simulink model "roll_pitch_pid_control_system1"  (R2016b)
settings: Solver=FixedStepDiscrete  StartTime=0.0  StopTime=inf  RelTol=1e-3
PostLoadFcn:
  | kFactor = 1.2;
  | 
  | KpRollAttitude = 0.630138625117681 / kFactor;
  | KiRollAttitude = 0.0552303199591522 / kFactor;
  | 
  | KpPitchAttitude = 0.630138625117681 / kFactor;
  | KiPitchAttitude = 0.0552303199591522 / kFactor;
  | 
  | KpRollRate = 1.31533836563383 / kFactor;
  | KiRollRate = 0.460338699849681 / kFactor;
  | 
  | KpPitchRate = 1.31533836563383 / kFactor;
  | KiPitchRate = 0.460338699849681 / kFactor;
  | 
  | KpYawRate = 1.31533836563383 / kFactor;
  | KiYawRate = 0.460338699849681 / kFactor;
undefined symbols (not defined in the file or in its folder): PX4_TUNE_ENUM, RGBLED_COLOR_ENUM, RGBLED_MODE_ENUM
libraries: pixhawk_slib_sensors_actuators x6, simulink x3
settings Model: SimulationMode=external  ExtModeTrigDuration=800  ExtModeArchiveFileName=EXT_mode_log  ExtModeArchiveDirName=C:\Pixhawk_Branch_Experiment\Ext_mode_bkgnd\Data_Logging  ExtModeAddSuffixToVar=on  ExtModeWriteAllDataToWs=on  ExtModeLogAll=off  Creator=Adam  LastModifiedBy=E6320
settings SolverCC: AutoInsertRateTranBlk=on
settings DataIOCC: LimitDataPoints=on  SaveFormat=Array
settings OptimizationCC: DefaultParameterBehavior=Inlined  LifeSpan=1  MaxStackSize=64
settings DebuggingCC: SolverPrmCheckMsg=warning  AllowSymbolicDim=off  SFUnexpectedBacktrackingDiag=warning  SFNoUnconditionalDefaultTransitionDiag=warning  SFExecutionAtInitializationDiag=none
settings HardwareCC: ProdBitPerPointer=32  ProdBitPerSizeT=32  ProdBitPerPtrDiffT=32  ProdLargestAtomicInteger=Long  ProdLargestAtomicFloat=Double  ProdWordSize=32  ProdHWDeviceType=ARM Compatible->ARM Cortex
settings ModelReferenceCC: PropagateSignalLabelsOutOfModel=off
settings RTWCC: SystemTargetFile=ert.tlc  HardwareBoard=Pixhawk PX4  TLCOptions=-aInlineSetEventsForThisBaseRateFcn=TLC_FALSE -aSuppressMultiTaskScheduler=TLC_FALSE -aRateBasedStepFcn=0  TemplateMakefile=ert_default_tmf  Description=Embedded Coder  GenerateReport=on  Toolchain=Pixhawk Toolchain  IncludeHyperlinkInReport=on  LaunchReport=on  GenerateTraceReport=on  GenerateTraceReportSl=on  GenerateTraceReportSf=on  GenerateTraceReportEml=on  GenerateCodeMetricsReport=on
settings CodeAppCC: IgnoreCustomStorageClasses=off
settings ERTTargetCC: CodeReplacementLibrary=GCC ARM Cortex-A9  ExtMode=on  ExtModeTransport=1  ExtModeMexFile=ext_serial_win32_comm  ExtModeMexArgs=1 7 115200 10  ERTCustomFileTemplate=PX4_codertarget_file_process.tlc  ConvertIfToSwitch=off  SuppressUnreachableDefaultCases=off
settings ConfigComp: CovMetricSettings=dw  CovHtmlReporting=on  CovSaveCumulativeToWorkspaceVar=on  CovSaveSingleToWorkspaceVar=on  CovExternalEMLEnable=off  CovSFcnEnable=off

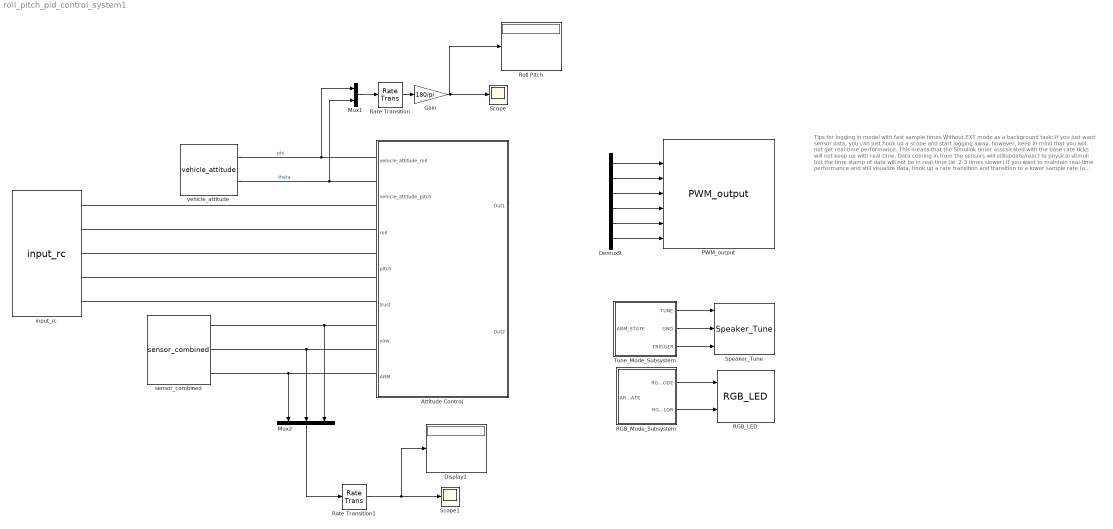
== system roll_pitch_pid_control_system1 ==
  note: Tips for logging in model with fast sample times
      |
      | Without EXT mode as a background task:
      | If you just want sensor data, you can just hook up a scope and start logging away, however, keep in mind that you will not get real-time performance. This means that the Simulink timer assosicated with the base-rate ticks will not keep up with real-time. Data coming in from the sensors will stillupdate/react to physical stimuli but the time stamp of data will not be in real-time (ie: 2-3 times slower)
      |
      | If you want to maintain real-time performance and still visualize data, hook up a rate transition and transition to a lower sample rate (a factor of 10 lower) and set the duration size to a value that will not cause the clock to slow down that much
      |
      | Recall that duration is the number of base-rate 'ticks' of data to give back. Sometimes if you set the duration too low data fails to come in for a specified sample rate. For instance, if we chose a duration value of 1:
      | 1 * 0.004 = 0.004 seconds worth of data
      | What will the lower sample (0.04s) scope show?
      | int( 0.004/0.04 ) = 0.. if we check the scope we see no data
      |
      | However, if we chose a duration value of 20
      | 400*0.004 = 1.6 seconds worth of data from base-rate
      | 1.60 / 0.04 = 40 points of data on the lower sample time scopes
      |
      | In other words, ensure the number of duration ticks gives you enough data
      | points to view on the lower sample rates, otherwise you wont see any data at all. Consult the documentation for more detail
      |
      | Using EXT mode with background task enabled
      |
      | This model has already been configured to use a background task and already uses a lot of the tips described in the above steps. With background tasking, the base-rate task is not encumbered by having to run external mode tasks at the same time, instead, EXT mode is now running in the background on another task being paced at 10 Hz. This can greatly help with real-time performance. Sometimes you may want to use the default behavior if you only have a single sample-time running at a slow rate - if you want data to come in faster or as fast as the model's sample-time then you'll want to use default behavior. On the other hand, if your model is running with multiple rates at varying speeds, you will want to pick the back-ground task option
  Attitude Control : Subsystem
  Demux9 : Demux  Outputs=6
  Display1 : Display
  Gain : Gain  Gain=180/pi
  Mux1 : Mux  Inputs=2
  Mux2 : Mux  Inputs=3
  PWM_output : pixhawk_slib_sensors_actuators/PWM_output  pwm_rate=400Hz  show_pwm1=on  show_pwm2=on  show_pwm3=on  show_pwm4=on  show_pwm5=on  show_pwm6=on  show_pwm7=off  show_pwm8=off
  RGB_LED : pixhawk_slib_sensors_actuators/RGB_LED
  RGB_Mode_Subsystem : Subsystem
  Rate Transition : RateTransition  OutPortSampleTime=0.04
  Rate Transition1 : RateTransition  OutPortSampleTime=0.04
  Roll Pitch : Display
  Scope : Scope
  Scope1 : Scope
  Speaker_Tune : pixhawk_slib_sensors_actuators/Speaker_Tune
  Tune_Mode_Subsystem : Subsystem
  input_rc : pixhawk_slib_sensors_actuators/input_rc  sampletime=1/250  channel1=on  channel2=on  channel3=on  channel4=on  channel5=on  channel6=off  channel7=off  channel8=off  ch_count=off  rssi=off  rc_failsafe=off  rc_lost=off  rc_inputsource=off
  sensor_combined : pixhawk_slib_sensors_actuators/sensor_combined  sampletime=1/250  show_mag=off  show_acc=off  show_gyro=on  show_baro=off  show_ts=off
  vehicle_attitude : pixhawk_slib_sensors_actuators/vehicle_attitude  sampletime=1/250  show_r=on  show_p=on  show_y=off  show_q=off
  wires:
  Demux9/6 -> PWM_output/7
  Demux9/5 -> PWM_output/6
  Demux9/4 -> PWM_output/5
  Demux9/2 -> PWM_output/3
  Demux9/3 -> PWM_output/4
  RGB_Mode_Subsystem/1(RGB_MODE) -> RGB_LED/1
  RGB_Mode_Subsystem/2(RGB_COLOR) -> RGB_LED/2
  Tune_Mode_Subsystem/1(TUNE) -> Speaker_Tune/1
  Tune_Mode_Subsystem/2(GND) -> Speaker_Tune/2
  Tune_Mode_Subsystem/3(TRIGGER) -> Speaker_Tune/3
  ? -> PWM_output/1, Tune_Mode_Subsystem/1(ARM_STATE), RGB_Mode_Subsystem/1(ARM_STATE)
  vehicle_attitude/1 -> Mux1/1  "phi"
  vehicle_attitude/2 -> Mux1/2  "theta"
  input_rc/1 -> ?
  input_rc/2 -> ?
  input_rc/3 -> ?
  input_rc/4 -> ?
  sensor_combined/1 -> Mux2/3
  sensor_combined/2 -> Mux2/2
  sensor_combined/3 -> Mux2/1
  ? -> Demux9/1
  Demux9/1 -> PWM_output/2
  input_rc/5 -> ?
  Mux1/1 -> Rate Transition/1
  Rate Transition/1 -> Gain/1
  Rate Transition1/1 -> Scope1/1, Display1/1
  Mux2/1 -> Rate Transition1/1
  Gain/1 -> Roll Pitch/1, Scope/1

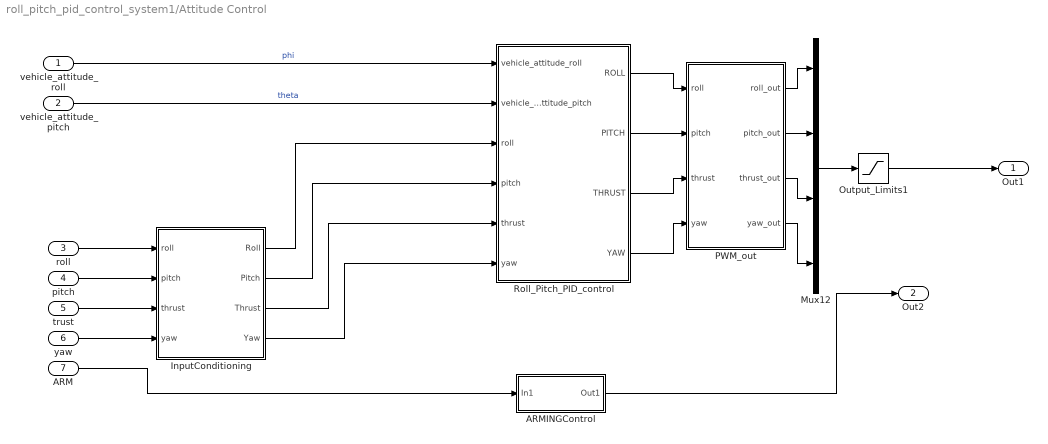
== system roll_pitch_pid_control_system1/Attitude Control ==
  vehicle_attitude_roll : Inport
  vehicle_attitude_pitch : Inport  Port=2
  roll : Inport  Port=3
  pitch : Inport  Port=4
  trust : Inport  Port=5
  yaw : Inport  Port=6
  ARM : Inport  Port=7
  ARMINGControl : Subsystem
  InputConditioning : Subsystem
  Mux12 : Mux
  Output_Limits1 : Saturate  UpperLimit=2000  LowerLimit=1000
  PWM_out : MATLAB Function  TreatAsAtomicUnit=on
  Roll_Pitch_PID_control : Subsystem
  Out1 : Outport
  Out2 : Outport  Port=2
  wires:
  vehicle_attitude_roll/1 -> Roll_Pitch_PID_control/1(vehicle_attitude_roll)  "phi"
  vehicle_attitude_pitch/1 -> Roll_Pitch_PID_control/2(vehicle_attitude_pitch)  "theta"
  ARM/1 -> ARMINGControl/1(In1)
  roll/1 -> InputConditioning/1(roll)
  pitch/1 -> InputConditioning/2(pitch)
  yaw/1 -> InputConditioning/4(yaw)
  trust/1 -> InputConditioning/3(thrust)
  ARMINGControl/1(Out1) -> Out2/1
  Output_Limits1/1 -> Out1/1
  InputConditioning/1(Roll) -> Roll_Pitch_PID_control/3(roll)
  InputConditioning/2(Pitch) -> Roll_Pitch_PID_control/4(pitch)
  InputConditioning/3(Thrust) -> Roll_Pitch_PID_control/5(thrust)
  InputConditioning/4(Yaw) -> Roll_Pitch_PID_control/6(yaw)
  Roll_Pitch_PID_control/4(YAW) -> PWM_out/4(yaw)
  Roll_Pitch_PID_control/3(THRUST) -> PWM_out/3(thrust)
  Roll_Pitch_PID_control/2(PITCH) -> PWM_out/2(pitch)
  Roll_Pitch_PID_control/1(ROLL) -> PWM_out/1(roll)
  PWM_out/1(roll_out) -> Mux12/1
  PWM_out/2(pitch_out) -> Mux12/2
  PWM_out/3(thrust_out) -> Mux12/3
  PWM_out/4(yaw_out) -> Mux12/4
  Mux12/1 -> Output_Limits1/1

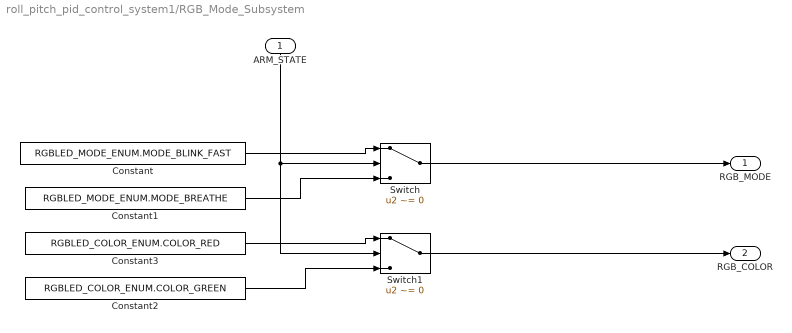
== system roll_pitch_pid_control_system1/RGB_Mode_Subsystem ==
  ARM_STATE : Inport
  Constant : Constant  Value=RGBLED_MODE_ENUM.MODE_BLINK_FAST  OutDataTypeStr=Enum: RGBLED_MODE_ENUM
  Constant1 : Constant  Value=RGBLED_MODE_ENUM.MODE_BREATHE  OutDataTypeStr=Enum: RGBLED_MODE_ENUM
  Constant2 : Constant  Value=RGBLED_COLOR_ENUM.COLOR_GREEN  OutDataTypeStr=Enum: RGBLED_COLOR_ENUM
  Constant3 : Constant  Value=RGBLED_COLOR_ENUM.COLOR_RED  OutDataTypeStr=Enum: RGBLED_COLOR_ENUM
  Switch : Switch  Criteria=u2 ~= 0  Threshold=1500  SampleTime=1/2
  Switch1 : Switch  Criteria=u2 ~= 0  Threshold=1500  SampleTime=1/2
  RGB_MODE : Outport
  RGB_COLOR : Outport  Port=2
  wires:
  ARM_STATE/1 -> Switch1/2, Switch/2
  Constant/1 -> Switch/1
  Constant1/1 -> Switch/3
  Switch/1 -> RGB_MODE/1
  Constant3/1 -> Switch1/1
  Constant2/1 -> Switch1/3
  Switch1/1 -> RGB_COLOR/1

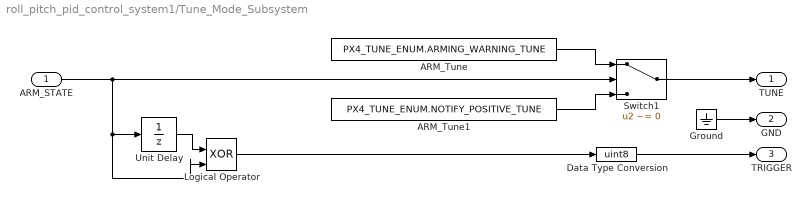
== system roll_pitch_pid_control_system1/Tune_Mode_Subsystem ==
  ARM_STATE : Inport
  ARM_Tune : Constant  Value=PX4_TUNE_ENUM.ARMING_WARNING_TUNE  OutDataTypeStr=Enum: PX4_TUNE_ENUM
  ARM_Tune1 : Constant  Value=PX4_TUNE_ENUM.NOTIFY_POSITIVE_TUNE  OutDataTypeStr=Enum: PX4_TUNE_ENUM
  Data Type Conversion : DataTypeConversion  OutDataTypeStr=uint8
  Ground : Ground
  Logical Operator : Logic  Operator=XOR  IconShape=distinctive  AllPortsSameDT=off  OutDataTypeStr=boolean
  Switch1 : Switch  Criteria=u2 ~= 0  Threshold=1500
  Unit Delay : UnitDelay  SampleTime=-1
  TUNE : Outport
  GND : Outport  Port=2
  TRIGGER : Outport  Port=3
  wires:
  Ground/1 -> GND/1
  Data Type Conversion/1 -> TRIGGER/1
  Switch1/1 -> TUNE/1
  ARM_Tune/1 -> Switch1/1
  ARM_Tune1/1 -> Switch1/3
  ARM_STATE/1 -> Logical Operator/2, Unit Delay/1, Switch1/2
  Unit Delay/1 -> Logical Operator/1
  Logical Operator/1 -> Data Type Conversion/1

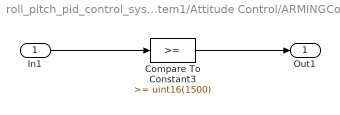
== system roll_pitch_pid_control_system1/Attitude Control/ARMINGControl ==
  In1 : Inport
  Compare To Constant3 : simulink/Logic and Bit Operations/Compare To Constant  relop=>=  const=uint16(1500)  OutDataTypeStr=boolean
  Out1 : Outport
  wires:
  Compare To Constant3/1 -> Out1/1
  In1/1 -> Compare To Constant3/1

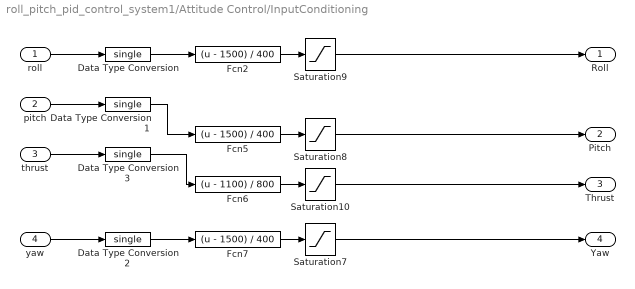
== system roll_pitch_pid_control_system1/Attitude Control/InputConditioning ==
  roll : Inport
  pitch : Inport  Port=2
  thrust : Inport  Port=3
  yaw : Inport  Port=4
  Data Type Conversion{,1..3} (4 alike) : DataTypeConversion  OutDataTypeStr=single
  Fcn2 : Fcn  Expr=(u - 1500) / 400
  Fcn5 : Fcn  Expr=(u - 1500) / 400
  Fcn6 : Fcn  Expr=(u - 1100) / 800
  Fcn7 : Fcn  Expr=(u - 1500) / 400
  Saturation10 : Saturate  UpperLimit=1  LowerLimit=0
  Saturation7 : Saturate  UpperLimit=1  LowerLimit=-1
  Saturation8 : Saturate  UpperLimit=1  LowerLimit=-1
  Saturation9 : Saturate  UpperLimit=1  LowerLimit=-1
  Roll : Outport
  Pitch : Outport  Port=2
  Thrust : Outport  Port=3
  Yaw : Outport  Port=4
  wires:
  Saturation10/1 -> Thrust/1
  Saturation7/1 -> Yaw/1
  Saturation8/1 -> Pitch/1
  Fcn6/1 -> Saturation10/1
  thrust/1 -> Data Type Conversion3/1
  Fcn2/1 -> Saturation9/1
  Fcn5/1 -> Saturation8/1
  Saturation9/1 -> Roll/1
  Fcn7/1 -> Saturation7/1
  yaw/1 -> Data Type Conversion2/1
  pitch/1 -> Data Type Conversion1/1
  roll/1 -> Data Type Conversion/1
  Data Type Conversion/1 -> Fcn2/1
  Data Type Conversion1/1 -> Fcn5/1
  Data Type Conversion2/1 -> Fcn7/1
  Data Type Conversion3/1 -> Fcn6/1

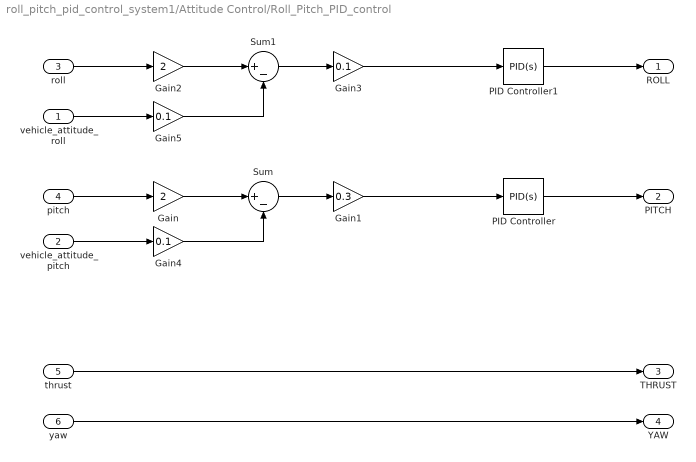
== system roll_pitch_pid_control_system1/Attitude Control/Roll_Pitch_PID_control ==
  vehicle_attitude_roll : Inport
  vehicle_attitude_pitch : Inport  Port=2
  roll : Inport  Port=3
  pitch : Inport  Port=4
  thrust : Inport  Port=5
  yaw : Inport  Port=6
  Gain : Gain  Gain=2
  Gain1 : Gain  Gain=0.3
  Gain2 : Gain  Gain=2
  Gain3 : Gain  Gain=0.1
  Gain4 : Gain  Gain=0.1
  Gain5 : Gain  Gain=0.1
  PID Controller : simulink/Continuous/PID Controller  Controller=PID  TimeDomain=Continuous-time  SampleTime=-1  IntegratorMethod=Forward Euler  FilterMethod=Forward Euler  Form=Parallel  UseFilter=on  ControllerParametersSource=internal  P=0.8  I=1  D=0.7  N=100  InitialConditionSource=internal  InitialConditionForIntegrator=0  InitialConditionForFilter=0  ExternalReset=none  LimitOutput=off  UpperSaturationLimit=inf  LowerSaturationLimit=-inf  LinearizeAsGain=on  AntiWindupMode=none  Kb=1  TrackingMode=off  Kt=1  PParamMin=[]  PParamMax=[]  IParamMin=[]  IParamMax=[]  DParamMin=[]  DParamMax=[]  NParamMin=[]  NParamMax=[]  KbParamMin=[]  KbParamMax=[]  KtParamMin=[]  KtParamMax=[]  POutMin=[]  POutMax=[]  IOutMin=[]  IOutMax=[]  DOutMin=[]  DOutMax=[]  NOutMin=[]  NOutMax=[]  KbOutMin=[]  KbOutMax=[]  KtOutMin=[]  KtOutMax=[]  IntegratorOutMin=[]  IntegratorOutMax=[]  FilterOutMin=[]  FilterOutMax=[]  SumOutMin=[]  SumOutMax=[]  SumI1OutMin=[]  SumI1OutMax=[]  SumI2OutMin=[]  SumI2OutMax=[]  SumI3OutMin=[]  SumI3OutMax=[]  SumDOutMin=[]  SumDOutMax=[]  SaturationOutMin=[]  SaturationOutMax=[]  IntegratorContinuousStateAttributes=''  IntegratorStateMustResolveToSignalObject=off  IntegratorRTWStateStorageClass=Auto  FilterContinuousStateAttributes=''  FilterStateMustResolveToSignalObject=off  FilterRTWStateStorageClass=Auto  DifferentiatorICPrevScaledInput=0  DifferentiatorOutMin=[]  DifferentiatorOutMax=[]
  PID Controller1 : simulink/Continuous/PID Controller  Controller=PID  TimeDomain=Continuous-time  SampleTime=-1  IntegratorMethod=Forward Euler  FilterMethod=Forward Euler  Form=Parallel  UseFilter=on  ControllerParametersSource=internal  P=0.8  I=1  D=0.7  N=100  InitialConditionSource=internal  InitialConditionForIntegrator=0  InitialConditionForFilter=0  ExternalReset=none  LimitOutput=off  UpperSaturationLimit=inf  LowerSaturationLimit=-inf  LinearizeAsGain=on  AntiWindupMode=none  Kb=1  TrackingMode=off  Kt=1  PParamMin=[]  PParamMax=[]  IParamMin=[]  IParamMax=[]  DParamMin=[]  DParamMax=[]  NParamMin=[]  NParamMax=[]  KbParamMin=[]  KbParamMax=[]  KtParamMin=[]  KtParamMax=[]  POutMin=[]  POutMax=[]  IOutMin=[]  IOutMax=[]  DOutMin=[]  DOutMax=[]  NOutMin=[]  NOutMax=[]  KbOutMin=[]  KbOutMax=[]  KtOutMin=[]  KtOutMax=[]  IntegratorOutMin=[]  IntegratorOutMax=[]  FilterOutMin=[]  FilterOutMax=[]  SumOutMin=[]  SumOutMax=[]  SumI1OutMin=[]  SumI1OutMax=[]  SumI2OutMin=[]  SumI2OutMax=[]  SumI3OutMin=[]  SumI3OutMax=[]  SumDOutMin=[]  SumDOutMax=[]  SaturationOutMin=[]  SaturationOutMax=[]  IntegratorContinuousStateAttributes=''  IntegratorStateMustResolveToSignalObject=off  IntegratorRTWStateStorageClass=Auto  FilterContinuousStateAttributes=''  FilterStateMustResolveToSignalObject=off  FilterRTWStateStorageClass=Auto  DifferentiatorICPrevScaledInput=0  DifferentiatorOutMin=[]  DifferentiatorOutMax=[]
  Sum : Sum  Inputs=|+-
  Sum1 : Sum  Inputs=|+-
  ROLL : Outport
  PITCH : Outport  Port=2
  THRUST : Outport  Port=3
  YAW : Outport  Port=4
  wires:
  pitch/1 -> Gain/1
  Gain/1 -> Sum/1
  vehicle_attitude_pitch/1 -> Gain4/1
  Sum/1 -> Gain1/1
  Gain1/1 -> PID Controller/1
  roll/1 -> Gain2/1
  Gain2/1 -> Sum1/1
  Sum1/1 -> Gain3/1
  Gain4/1 -> Sum/2
  vehicle_attitude_roll/1 -> Gain5/1
  Gain5/1 -> Sum1/2
  Gain3/1 -> PID Controller1/1
  PID Controller1/1 -> ROLL/1
  PID Controller/1 -> PITCH/1
  thrust/1 -> THRUST/1
  yaw/1 -> YAW/1

== matlab function roll_pitch_pid_control_system1/Attitude Control/PWM_out ==
  data: roll input; roll_out output; pitch input; thrust input; yaw input; pitch_out output; thrust_out output; yaw_out output
function [roll_out,pitch_out,thrust_out,yaw_out] = fcn(roll,pitch,thrust,yaw)
roll_out=uint16(1500+(roll)*400);
pitch_out=uint16(1500+(pitch)*400);
thrust_out=uint16(1100+(thrust)*800);
yaw=uint16(1500+(thrust)*400);
